simulink model "structure"  (R2015a)
settings: Solver=FixedStepDiscrete  StartTime=0.0  StopTime=10.0  FixedStep=delta_t  RelTol=1e-3
undefined symbols (not defined in the file): ca1, ca2, ca3, ca4, cb, D, delta_t, I, Inv_I, m, S, S_pinv, sa1, sa2, sa3, sa4, sb
settings Model: Creator=Kerianne  LastModifiedBy=Kerianne
settings DataIOCC: SaveFormat=Structure
settings OptimizationCC: InlineParams=on  ExpressionDepthLimit=2147483647
settings DebuggingCC: UnderspecifiedInitializationDetection=Classic  MergeDetectMultiDrivingBlocksExec=none  SolverPrmCheckMsg=warning  StateNameClashWarn=warning

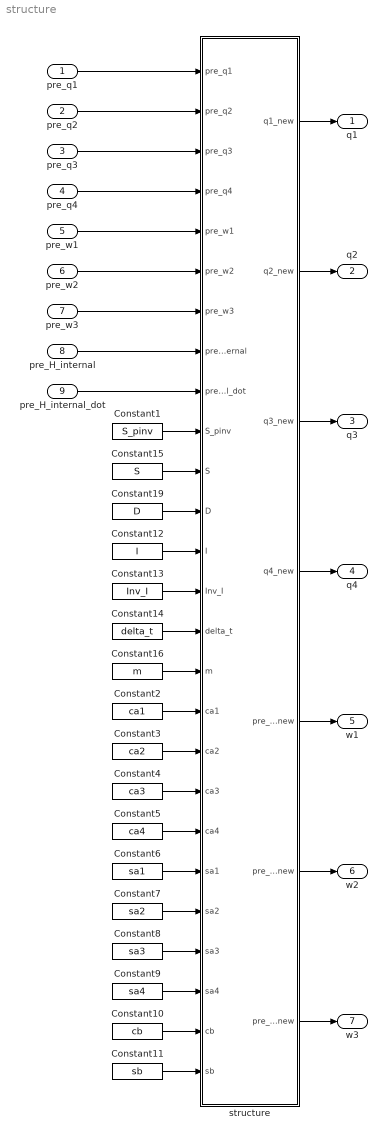
== system structure ==
  pre_q1 : Inport
  pre_q2 : Inport  Port=2
  pre_q3 : Inport  Port=3
  pre_q4 : Inport  Port=4
  pre_w1 : Inport  Port=5
  pre_w2 : Inport  Port=6
  pre_w3 : Inport  Port=7
  pre_H_internal : Inport  Port=8  PortDimensions=3
  pre_H_internal_dot : Inport  Port=9  PortDimensions=3
  Constant1 : Constant  Value=S_pinv
  Constant10 : Constant  Value=cb
  Constant11 : Constant  Value=sb
  Constant12 : Constant  Value=I
  Constant13 : Constant  Value=Inv_I
  Constant14 : Constant  Value=delta_t
  Constant15 : Constant  Value=S
  Constant16 : Constant  Value=m
  Constant19 : Constant  Value=D
  Constant2 : Constant  Value=ca1
  Constant3 : Constant  Value=ca2
  Constant4 : Constant  Value=ca3
  Constant5 : Constant  Value=ca4
  Constant6 : Constant  Value=sa1
  Constant7 : Constant  Value=sa2
  Constant8 : Constant  Value=sa3
  Constant9 : Constant  Value=sa4
  structure : MATLAB Function  TreatAsAtomicUnit=on
  q1 : Outport
  q2 : Outport  Port=2
  q3 : Outport  Port=3
  q4 : Outport  Port=4
  w1 : Outport  Port=5
  w2 : Outport  Port=6
  w3 : Outport  Port=7
  wires:
  structure/1(q1_new) -> q1/1
  structure/2(q2_new) -> q2/1
  structure/3(q3_new) -> q3/1
  structure/4(q4_new) -> q4/1
  structure/5(pre_w1_new) -> w1/1
  structure/6(pre_w2_new) -> w2/1
  structure/7(pre_w3_new) -> w3/1
  Constant14/1 -> structure/15(delta_t)
  Constant19/1 -> structure/12(D)
  Constant12/1 -> structure/13(I)
  Constant13/1 -> structure/14(Inv_I)
  pre_w3/1 -> structure/7(pre_w3)
  pre_w2/1 -> structure/6(pre_w2)
  pre_w1/1 -> structure/5(pre_w1)
  pre_q4/1 -> structure/4(pre_q4)
  pre_q3/1 -> structure/3(pre_q3)
  pre_q2/1 -> structure/2(pre_q2)
  pre_q1/1 -> structure/1(pre_q1)
  Constant16/1 -> structure/16(m)
  pre_H_internal_dot/1 -> structure/9(pre_H_internal_dot)
  pre_H_internal/1 -> structure/8(pre_H_internal)
  Constant1/1 -> structure/10(S_pinv)
  Constant6/1 -> structure/21(sa1)
  Constant5/1 -> structure/20(ca4)
  Constant4/1 -> structure/19(ca3)
  Constant3/1 -> structure/18(ca2)
  Constant2/1 -> structure/17(ca1)
  Constant11/1 -> structure/26(sb)
  Constant10/1 -> structure/25(cb)
  Constant9/1 -> structure/24(sa4)
  Constant8/1 -> structure/23(sa3)
  Constant7/1 -> structure/22(sa2)
  Constant15/1 -> structure/11(S)

== matlab function structure/structure ==
  data: pre_q1 input; pre_q2 input; pre_q3 input; pre_q4 input; pre_w1 input; pre_w2 input; pre_w3 input; pre_H_internal input; pre_H_internal_dot input; S_pinv input; S input; q1_new output; D input; I input; Inv_I input; delta_t input; q2_new output; q3_new output; q4_new output; pre_w1_new output; pre_w2_new output; pre_w3_new output; m input; ca1 input; ca2 input; ca3 input; ca4 input; sa1 input; sa2 input; sa3 input; sa4 input; cb input; sb input
function  [q1_new,q2_new,q3_new,q4_new,pre_w1_new,pre_w2_new,pre_w3_new]= fcn(pre_q1,pre_q2,pre_q3,pre_q4,pre_w1,pre_w2,pre_w3,pre_H_internal,pre_H_internal_dot,S_pinv,S,D,I,Inv_I,delta_t,m,ca1,ca2,ca3,ca4,sa1,sa2,sa3,sa4,cb,sb)
% Structure
% Author: Kerianne Gross, kerianne.gross@us.af.mil
% Date Update: 7 May 2015

% This file updates the state of the spacecraft structure including it's
% quaternion orienation and angular velocity, given its previous state,
% angular momentum, and the change in angular momentum from the RWA.

% ca1,ca2,ca3,ca4,sa1,sa2,sa3,sa4,cb,sb
q = [pre_q1;pre_q2;pre_q3;pre_q4];
omega = [pre_w1;pre_w2;pre_w3];
pre_psi = S_pinv*pre_H_internal;  
psi_1 = pre_psi(1);
psi_2 = pre_psi(2);
psi_3 = pre_psi(3);
psi_4 = pre_psi(4);
psi_dot = S_pinv*pre_H_internal_dot;

x = [pre_q1;pre_q2;pre_q3;pre_q4;pre_w1;pre_w2;pre_w3;psi_1;psi_2;psi_3;psi_4];

% Cubsat State derivative (not using ODE 45)
A11 = zeros(4,4);
A12 = 0.5*[ q(4) -q(3)  q(2);...
            q(3)  q(4) -q(1);...
           -q(2)  q(1)  q(4);...
           -q(1) -q(2) -q(3)];
A13 = zeros(4,4);
A21 = zeros(3,4);
A22 = -Inv_I*skew([omega(1) omega(2) omega(3)])*I;
A23 = -Inv_I*skew([omega(1) omega(2) omega(3)])*S;
A31 = zeros(4,4); A32 = zeros(4,3); 
A33 = zeros(4,4); %% use this for no magnetic torque
m = [0;0;0]; %% use this for no magnetic torque

A = [A11 A12 A13; A21 A22 A23; A31 A32 A33];
B = [zeros(4,3); Inv_I; zeros(4,3)];
C = [zeros(7,4);eye(4,4)];
 
x_dot = A*x - B*S*psi_dot + B*m + C*psi_dot;
    
x_new = x + x_dot*delta_t;
q1_new = x_new(1);
q2_new = x_new(2);
q3_new = x_new(3);
q4_new = x_new(4);
pre_w1_new = x_new(5);
pre_w2_new = x_new(6);
pre_w3_new = x_new(7);
